simulink model "lab4"  (R2019b)
settings: Solver=VariableStepAuto  StartTime=0.0  StopTime=10.0  RelTol=1e-3
libraries: simulink x3
settings Model: NumberOfSteps=2  SnapshotBufferSize=20  SnapshotInterval=20  Creator=1  LastModifiedBy=1

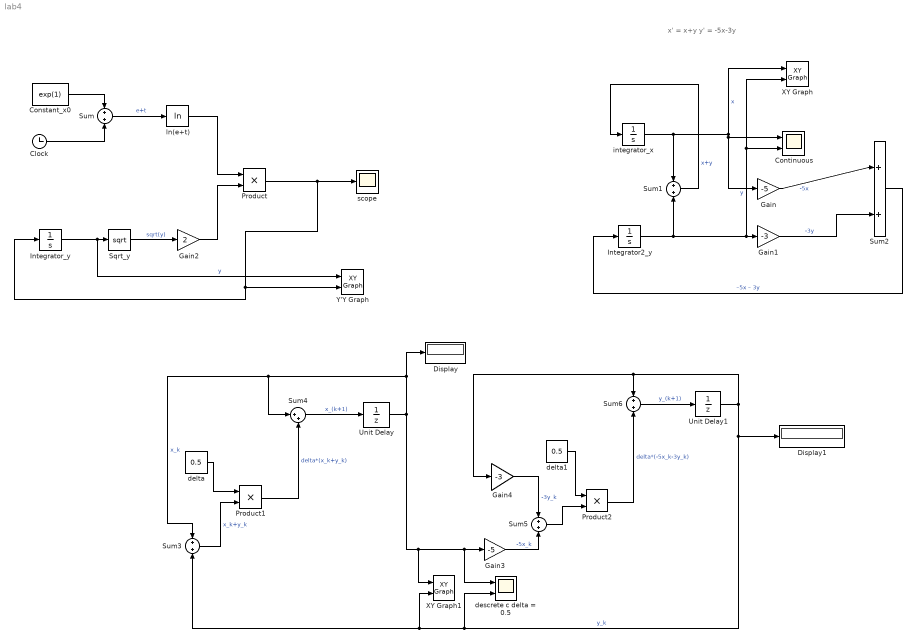
== system lab4 ==
  note: x' = x+y
      | y' = -5x-3y
  Clock : Clock
  Constant_x0 : Constant  Value=exp(1)
  Continuous : Scope  NumInputPorts=2
  Display : Display
  Display1 : Display
  Gain : Gain  Gain=-5
  Gain1 : Gain  Gain=-3
  Gain2 : Gain  Gain=2
  Gain3 : Gain  Gain=-5
  Gain4 : Gain  Gain=-3
  Integrator2_y : Integrator
  Integrator_y : Integrator  InitialCondition=1
  Product : Product
  Product1 : Product
  Product2 : Product
  Sqrt_y : Sqrt  SaturateOnIntegerOverflow=on
  Sum{,1,3,5..6} (5 alike) : Sum
  Sum2 : Sum  Inputs=|++
  Sum4 : Sum  Inputs=|++
  Unit Delay : UnitDelay  InitialCondition=1  SampleTime=-1  HasFrameUpgradeWarning=on
  Unit Delay1 : UnitDelay  SampleTime=-1  HasFrameUpgradeWarning=on
  XY Graph : simulink/Sinks/XY Graph  xmin=-1  xmax=3  ymin=-3  ymax=1  st=-1
  XY Graph1 : simulink/Sinks/XY Graph  xmin=-1  xmax=3  ymin=-3  ymax=1  st=-1
  Y'Y Graph : simulink/Sinks/XY Graph  xmin=-3  xmax=25  ymin=-3  ymax=18  st=-1
  delta : Constant  Value=0.5
  delta1 : Constant  Value=0.5
  descrete c delta = 0.5 : Scope  NumInputPorts=2
  integrator_x : Integrator  InitialCondition=1
  "ln(e+t) " : Math  Operator=log  SignedPower=off  SaturateOnIntegerOverflow=on
  scope : Scope
  wires:
  Constant_x0/1 -> Sum/1
  Clock/1 -> Sum/2
  Sum/1 -> "ln(e+t) "/1  "e+t"
  Integrator_y/1 -> Y'Y Graph/1, Sqrt_y/1  "y"
  Sqrt_y/1 -> Gain2/1  "sqrt(y)"
  Gain2/1 -> Product/2
  "ln(e+t) "/1 -> Product/1
  Product/1 -> Integrator_y/1, Y'Y Graph/2, scope/1
  integrator_x/1 -> Sum1/1, Continuous/1, Gain/1, XY Graph/1  "x"
  Integrator2_y/1 -> XY Graph/2, Continuous/2, Gain1/1, Sum1/2  "y"
  Sum1/1 -> integrator_x/1  "x+y"
  Gain/1 -> Sum2/1  "-5x"
  Gain1/1 -> Sum2/2  "-3y"
  Sum2/1 -> Integrator2_y/1  "–5x – 3y"
  Sum3/1 -> Product1/2  "x_k​+y_k"
  delta/1 -> Product1/1
  Product1/1 -> Sum4/2  "delta*(x_k+y_k)"
  Sum4/1 -> Unit Delay/1  "x_(k+1)"
  Unit Delay/1 -> XY Graph1/1, descrete c delta = 0.5/1, Gain3/1, Display/1, Sum4/1, Sum3/1  "x_k"
  Gain3/1 -> Sum5/2  "-5x_k"
  Gain4/1 -> Sum5/1  "-3y_k"
  Sum5/1 -> Product2/2
  delta1/1 -> Product2/1
  Product2/1 -> Sum6/2  "delta*(-5x_k-3y_k)"
  Sum6/1 -> Unit Delay1/1  "y_(k+1)"
  Unit Delay1/1 -> Gain4/1, Sum6/1, Display1/1, descrete c delta = 0.5/2, XY Graph1/2, Sum3/2  "y_k"
